simulink model "anti_interference"  (Simulink 7.2)
settings: Solver=ode45  StartTime=0.0  StopTime=0.02  RelTol=1e-3
undefined symbols (not defined in the file): get
libraries: dspbuff3 x24, dspxfrm3 x8, simulink x6, dspsigops x4, dspobslib x4, dspsnks4 x1
settings Model: Creator=Administrator  LastModifiedBy=Administrator

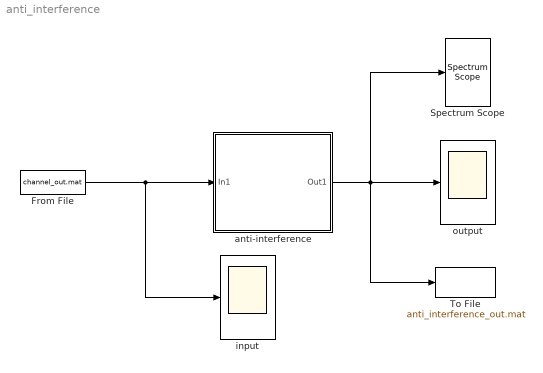
== system anti_interference ==
  From File : FromFile  FileName=channel_out.mat  SampleTime=1/5.1e6
  Spectrum Scope : dspsnks4/Spectrum Scope  DialogController=dspdialog.SpectrumScope  DialogControllerArgs=DataTag0  SystemSampleTime=-1  ScopeProperties=on  Domain=Frequency  HorizSpan=1  UseBuffer=on  BufferSize=2048  Overlap=64  inpFftLenInherit=off  FFTlength=128  numAvg=2  DisplayProperties=off  AxisGrid=on  Memory=off  FrameNumber=on  AxisLegend=off  AxisZoom=off  OpenScopeAtSimStart=on  OpenScopeImmediately=off  FigPos=get(0,'defaultfigureposition')  AxisProperties=off  XUnits=Hertz  XRange=[0...Fs/2]  XDisplay=0  InheritXIncr=on  XIncr=1.0  XLabel=Samples  XLimit=Auto  YUnits=dB  XMax=1  XMin=0  YLabel=Magnitude-squared, dB  LineProperties=off  wintypeSpecScope=Hann  RsSpecScope=50  betaSpecScope=5  winsampSpecScope=Periodic
      settings: YMin=-21.2867739282485  YMax=15.4884772920994
  To File : ToFile  Filename=anti_interference_out.mat
  anti-interference : Subsystem
  input : Scope
  output : Scope
  wires:
  From File/1 -> anti-interference/1(In1), input/1
  anti-interference/1(Out1) -> output/1, Spectrum Scope/1, To File/1

== system anti_interference/anti-interference ==
  In1 : Inport  OutDataType=sfix(16)  OutScaling=2^0
  Add1 : Sum  Inputs=++++  OutDataType=sfix(16)  OutScaling=2^-10
  Scope : Scope  NumInputPorts=5
      settings: YMin=-5~-5~-5~-5~-5  YMax=5~5~5~5~5  SaveName=ScopeData2
  firstroad : Subsystem
  fourthroad : Subsystem
  secondroad : Subsystem
  thirdroad : Subsystem
  Out1 : Outport  OutDataType=sfix(16)  OutScaling=2^0
  wires:
  firstroad/1(Out1) -> Add1/1, Scope/1
  secondroad/1(Out1) -> Add1/2, Scope/2
  thirdroad/1(Out1) -> Add1/3, Scope/3
  fourthroad/1(Out1) -> Add1/4, Scope/4
  In1/1 -> firstroad/1(In1), secondroad/1(In1), thirdroad/1(In1), fourthroad/1(In1)
  Add1/1 -> Out1/1, Scope/5

== system anti_interference/anti-interference/firstroad ==
  In1 : Inport  OutDataType=sfix(16)  OutScaling=2^0
  Complex to Magnitude-Angle : ComplexToMagnitudeAngle
  fft trans : Subsystem
  inteference_delieve : Subsystem
  inverse_convertion : Subsystem  Orientation=left
  threshold : Subsystem
  Out1 : Outport  Orientation=left  OutDataType=sfix(16)  OutScaling=2^0
  wires:
  fft trans/1(Out1) -> Complex to Magnitude-Angle/1
  Complex to Magnitude-Angle/1 -> threshold/1(In1), inteference_delieve/1(In1)
  Complex to Magnitude-Angle/2 -> inverse_convertion/1(In1)
  inteference_delieve/1(Out1) -> inverse_convertion/2(In2)
  threshold/1(Out1) -> inteference_delieve/2(In2)
  In1/1 -> fft trans/1(In1)
  inverse_convertion/1(Out1) -> Out1/1

== system anti_interference/anti-interference/fourthroad ==
  In1 : Inport  OutDataType=sfix(16)  OutScaling=2^0
  Complex to Magnitude-Angle : ComplexToMagnitudeAngle
  all : Subsystem
  inteference_delieve : Subsystem
  inverse_convertion : Subsystem  Orientation=left
  threshold : Subsystem
  Out1 : Outport  Orientation=left  OutDataType=sfix(16)  OutScaling=2^0
  wires:
  inverse_convertion/1(Out1) -> Out1/1
  In1/1 -> all/1(In1)
  threshold/1(Out1) -> inteference_delieve/2(In2)
  inteference_delieve/1(Out1) -> inverse_convertion/2(In2)
  Complex to Magnitude-Angle/2 -> inverse_convertion/1(In1)
  Complex to Magnitude-Angle/1 -> inteference_delieve/1(In1), threshold/1(In1)
  all/1(Out1) -> Complex to Magnitude-Angle/1

== system anti_interference/anti-interference/secondroad ==
  In1 : Inport  OutDataType=sfix(16)  OutScaling=2^0
  Complex to Magnitude-Angle : ComplexToMagnitudeAngle
  all : Subsystem
  inteference_delieve : Subsystem
  inverse_convertion : Subsystem  Orientation=left
  threshold : Subsystem
  Out1 : Outport  Orientation=left  OutDataType=sfix(16)  OutScaling=2^0
  wires:
  inverse_convertion/1(Out1) -> Out1/1
  In1/1 -> all/1(In1)
  threshold/1(Out1) -> inteference_delieve/2(In2)
  inteference_delieve/1(Out1) -> inverse_convertion/2(In2)
  Complex to Magnitude-Angle/2 -> inverse_convertion/1(In1)
  Complex to Magnitude-Angle/1 -> inteference_delieve/1(In1), threshold/1(In1)
  all/1(Out1) -> Complex to Magnitude-Angle/1

== system anti_interference/anti-interference/thirdroad ==
  In1 : Inport  OutDataType=sfix(16)  OutScaling=2^0
  Complex to Magnitude-Angle : ComplexToMagnitudeAngle
  all : Subsystem
  inteference_delieve : Subsystem
  inverse_convertion : Subsystem  Orientation=left
  threshold : Subsystem
  Out1 : Outport  Orientation=left  OutDataType=sfix(16)  OutScaling=2^0
  wires:
  all/1(Out1) -> Complex to Magnitude-Angle/1
  Complex to Magnitude-Angle/1 -> threshold/1(In1), inteference_delieve/1(In1)
  Complex to Magnitude-Angle/2 -> inverse_convertion/1(In1)
  inteference_delieve/1(Out1) -> inverse_convertion/2(In2)
  threshold/1(Out1) -> inteference_delieve/2(In2)
  In1/1 -> all/1(In1)
  inverse_convertion/1(Out1) -> Out1/1

== system anti_interference/anti-interference/firstroad/fft trans ==
  In1 : Inport  OutDataType=sfix(16)  OutScaling=2^0
  Buffer : dspbuff3/Buffer  N=8192  V=0  ic=0
  FFT1 : dspxfrm3/FFT  DialogController=dspDDGCreate  DialogControllerArgs=DataTag1  CompMethod=Table lookup  TableOpt=NEW  TableOptActive=Speed  BitRevOrder=off  InheritFFTLength=on  FFTLength=64  SkipNorm=off  roundingMode=Floor  overflowMode=off
  Window Function : dspsigops/Window Function  DialogController=dspDDGCreate  DialogControllerArgs=DataTag2  winmode=Apply window to input  wintype=Chebyshev  sampmode=Continuous  samptime=1  N=64  Rs=80  beta=10  winsamp=Symmetric  UserWindow=hamming  OptParams=off  UserParams={'symmetric'}  dataType=double  isSigned=on  wordLen=16  udDataType=sfix(16)  fracBitsMode=Best precision  numFracBits=15  roundingMode=Floor  overflowMode=off  numSidelobes=4  sidelobeLevel=-30
  Out1 : Outport  OutDataType=sfix(16)  OutScaling=2^0
  wires:
  Buffer/1 -> Window Function/1
  FFT1/1 -> Out1/1
  In1/1 -> Buffer/1
  Window Function/1 -> FFT1/1

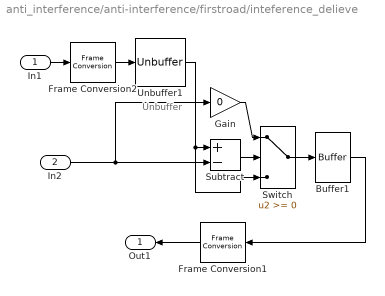
== system anti_interference/anti-interference/firstroad/inteference_delieve ==
  note: Unbuffer
  In1 : Inport  OutDataType=sfix(16)  OutScaling=2^0
  In2 : Inport  Port=2  OutDataType=sfix(16)  OutScaling=2^0
  Buffer1 : dspbuff3/Buffer  N=8192  V=0  ic=0
  Frame Conversion1 : FrameConversion  Orientation=left  OutFrame=Sample-based
  Frame Conversion2 : FrameConversion
  Gain : Gain  Gain=0  ParameterDataType=sfix(16)  ParameterScaling=2^0  OutDataType=sfix(16)  OutScaling=2^0
  Subtract : Sum  Inputs=+-  OutDataType=sfix(16)  OutScaling=2^-10
  Switch : Switch
  Unbuffer1 : dspbuff3/Unbuffer  ic=0
  Out1 : Outport  Orientation=left  OutDataType=sfix(16)  OutScaling=2^0
  wires:
  Unbuffer1/1 -> Subtract/1, Switch/3
  In2/1 -> Subtract/2, Gain/1
  Subtract/1 -> Switch/2
  Gain/1 -> Switch/1
  Switch/1 -> Buffer1/1
  In1/1 -> Frame Conversion2/1
  Frame Conversion2/1 -> Unbuffer1/1
  Frame Conversion1/1 -> Out1/1
  Buffer1/1 -> Frame Conversion1/1

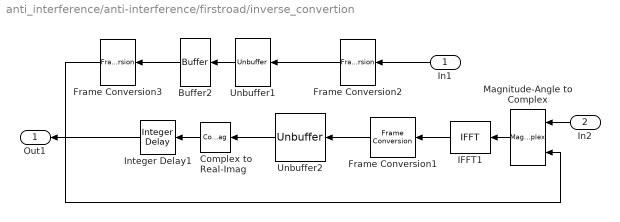
== system anti_interference/anti-interference/firstroad/inverse_convertion ==
  In1 : Inport  Orientation=left  OutDataType=sfix(16)  OutScaling=2^0
  In2 : Inport  Orientation=left  Port=2  OutDataType=sfix(16)  OutScaling=2^0
  Buffer2 : dspbuff3/Buffer  Orientation=left  N=8192  V=0  ic=0
  Complex to Real-Imag : ComplexToRealImag  Orientation=left  Output=Real
  Frame Conversion1 : FrameConversion  Orientation=left
  Frame Conversion2 : FrameConversion  Orientation=left
  Frame Conversion3 : FrameConversion  Orientation=left  OutFrame=Sample-based
  IFFT1 : dspxfrm3/IFFT  Orientation=left  DialogController=dspDDGCreate  DialogControllerArgs=DataTag3  CompMethod=Table lookup  TableOpt=NEW  TableOptActive=Speed  BitRevOrder=off  cs_in=off  SkipNorm=on  InheritFFTLength=on  FFTLength=64  mode=Complex  outSamplingMode=Sample based  roundingMode=Floor  overflowMode=off
  Integer Delay1 : simulink/Discrete/Integer Delay  Orientation=left  vinit=0.0  samptime=-1  NumDelays=6144
  Magnitude-Angle to Complex : MagnitudeAngleToComplex  Orientation=left
  Unbuffer1 : dspbuff3/Unbuffer  Orientation=left  ic=0
  Unbuffer2 : dspbuff3/Unbuffer  Orientation=left  ic=0
  Out1 : Outport  Orientation=left  OutDataType=sfix(16)  OutScaling=2^0
  wires:
  Frame Conversion2/1 -> Unbuffer1/1
  Unbuffer1/1 -> Buffer2/1
  Buffer2/1 -> Frame Conversion3/1
  Magnitude-Angle to Complex/1 -> IFFT1/1
  Unbuffer2/1 -> Complex to Real-Imag/1
  Frame Conversion3/1 -> Magnitude-Angle to Complex/2
  Complex to Real-Imag/1 -> Integer Delay1/1
  In1/1 -> Frame Conversion2/1
  In2/1 -> Magnitude-Angle to Complex/1
  IFFT1/1 -> Frame Conversion1/1
  Frame Conversion1/1 -> Unbuffer2/1
  Integer Delay1/1 -> Out1/1

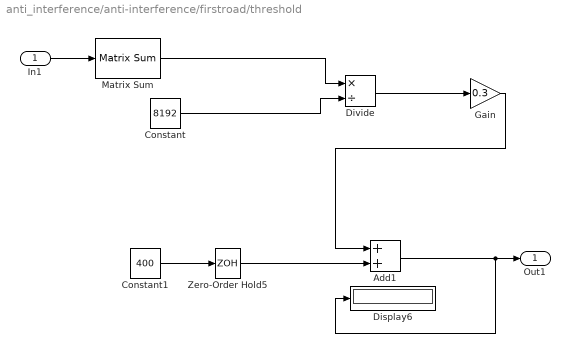
== system anti_interference/anti-interference/firstroad/threshold ==
  In1 : Inport  OutDataType=sfix(16)  OutScaling=2^0
  Add1 : Sum  OutDataType=sfix(16)  OutScaling=2^-10
  Constant : Constant  Value=8192  OutDataType=sfix(16)  OutScaling=2^0
  Constant1 : Constant  Value=400  OutDataType=sfix(16)  OutScaling=2^0
  Display6 : Display
  Divide : Product  Inputs=*/  OutDataType=sfix(16)  OutScaling=2^-10
  Gain : Gain  Gain=0.3  ParameterDataType=sfix(16)  ParameterScaling=2^0  OutDataType=sfix(16)  OutScaling=2^0
  Matrix Sum : dspobslib/Matrix Sum  DialogController=dspDDGCreate  DialogControllerArgs=DataTag4  Dim=Columns  roundingMode=Floor  overflowMode=off
  Zero-Order Hold5 : ZeroOrderHold  SampleTime=1/5.1e6
  Out1 : Outport  OutDataType=sfix(16)  OutScaling=2^0
  wires:
  Matrix Sum/1 -> Divide/1
  Divide/1 -> Gain/1
  Gain/1 -> Add1/1
  Add1/1 -> Display6/1, Out1/1
  In1/1 -> Matrix Sum/1
  Constant1/1 -> Zero-Order Hold5/1
  Constant/1 -> Divide/2
  Zero-Order Hold5/1 -> Add1/2

== system anti_interference/anti-interference/fourthroad/all ==
  In1 : Inport  OutDataType=sfix(16)  OutScaling=2^0
  Buffer1 : dspbuff3/Buffer  N=8192  V=0  ic=0
  FFT : dspxfrm3/FFT  DialogController=dspDDGCreate  DialogControllerArgs=DataTag5  CompMethod=Table lookup  TableOpt=NEW  TableOptActive=Speed  BitRevOrder=off  InheritFFTLength=on  FFTLength=64  SkipNorm=off  roundingMode=Floor  overflowMode=off
  Integer Delay : simulink/Discrete/Integer Delay  vinit=0.0  samptime=-1  NumDelays=6144
  Window Function1 : dspsigops/Window Function  DialogController=dspDDGCreate  DialogControllerArgs=DataTag6  winmode=Apply window to input  wintype=Chebyshev  sampmode=Continuous  samptime=1  N=64  Rs=80  beta=10  winsamp=Symmetric  UserWindow=hamming  OptParams=off  UserParams={'symmetric'}  dataType=double  isSigned=on  wordLen=16  udDataType=sfix(16)  fracBitsMode=Best precision  numFracBits=15  roundingMode=Floor  overflowMode=off  numSidelobes=4  sidelobeLevel=-30
  Out1 : Outport  OutDataType=sfix(16)  OutScaling=2^0
  wires:
  In1/1 -> Buffer1/1
  Buffer1/1 -> Integer Delay/1
  Integer Delay/1 -> Window Function1/1
  Window Function1/1 -> FFT/1
  FFT/1 -> Out1/1

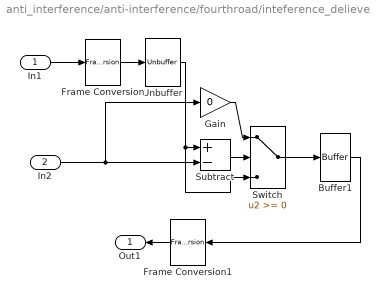
== system anti_interference/anti-interference/fourthroad/inteference_delieve ==
  In1 : Inport  OutDataType=sfix(16)  OutScaling=2^0
  In2 : Inport  Port=2  OutDataType=sfix(16)  OutScaling=2^0
  Buffer1 : dspbuff3/Buffer  N=8192  V=0  ic=0
  Frame Conversion : FrameConversion
  Frame Conversion1 : FrameConversion  Orientation=left  OutFrame=Sample-based
  Gain : Gain  Gain=0  ParameterDataType=sfix(16)  ParameterScaling=2^0  OutDataType=sfix(16)  OutScaling=2^0
  Subtract : Sum  Inputs=+-  OutDataType=sfix(16)  OutScaling=2^-10
  Switch : Switch
  Unbuffer : dspbuff3/Unbuffer  ic=0
  Out1 : Outport  Orientation=left  OutDataType=sfix(16)  OutScaling=2^0
  wires:
  Frame Conversion1/1 -> Out1/1
  In1/1 -> Frame Conversion/1
  Buffer1/1 -> Frame Conversion1/1
  Switch/1 -> Buffer1/1
  Gain/1 -> Switch/1
  Subtract/1 -> Switch/2
  In2/1 -> Gain/1, Subtract/2
  Frame Conversion/1 -> Unbuffer/1
  Unbuffer/1 -> Switch/3, Subtract/1

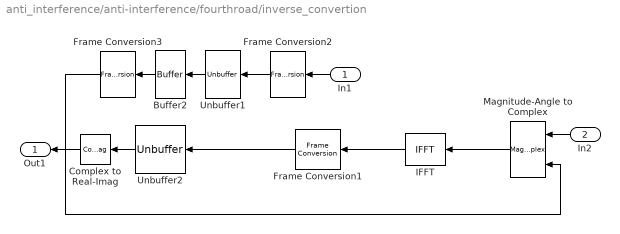
== system anti_interference/anti-interference/fourthroad/inverse_convertion ==
  In1 : Inport  Orientation=left  OutDataType=sfix(16)  OutScaling=2^0
  In2 : Inport  Orientation=left  Port=2  OutDataType=sfix(16)  OutScaling=2^0
  Buffer2 : dspbuff3/Buffer  Orientation=left  N=8192  V=0  ic=0
  Complex to Real-Imag : ComplexToRealImag  Orientation=left  Output=Real
  Frame Conversion1 : FrameConversion  Orientation=left
  Frame Conversion2 : FrameConversion  Orientation=left
  Frame Conversion3 : FrameConversion  Orientation=left  OutFrame=Sample-based
  IFFT : dspxfrm3/IFFT  Orientation=left  DialogController=dspDDGCreate  DialogControllerArgs=DataTag7  CompMethod=Table lookup  TableOpt=NEW  TableOptActive=Speed  BitRevOrder=off  cs_in=off  SkipNorm=on  InheritFFTLength=on  FFTLength=64  mode=Complex  outSamplingMode=Sample based  roundingMode=Floor  overflowMode=off
  Magnitude-Angle to Complex : MagnitudeAngleToComplex  Orientation=left
  Unbuffer1 : dspbuff3/Unbuffer  Orientation=left  ic=0
  Unbuffer2 : dspbuff3/Unbuffer  Orientation=left  ic=0
  Out1 : Outport  Orientation=left  OutDataType=sfix(16)  OutScaling=2^0
  wires:
  In2/1 -> Magnitude-Angle to Complex/1
  In1/1 -> Frame Conversion2/1
  Complex to Real-Imag/1 -> Out1/1
  Frame Conversion3/1 -> Magnitude-Angle to Complex/2
  Unbuffer2/1 -> Complex to Real-Imag/1
  Magnitude-Angle to Complex/1 -> IFFT/1
  Buffer2/1 -> Frame Conversion3/1
  Unbuffer1/1 -> Buffer2/1
  Frame Conversion2/1 -> Unbuffer1/1
  IFFT/1 -> Frame Conversion1/1
  Frame Conversion1/1 -> Unbuffer2/1

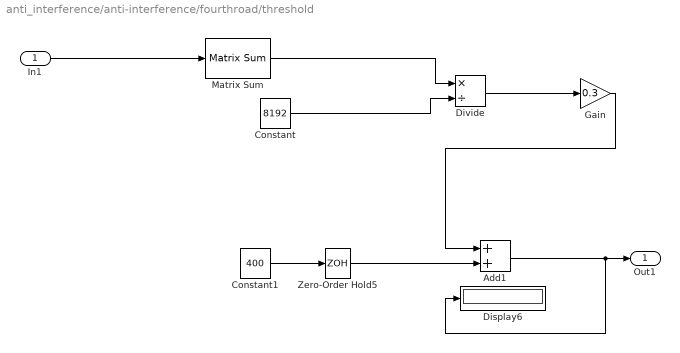
== system anti_interference/anti-interference/fourthroad/threshold ==
  In1 : Inport  OutDataType=sfix(16)  OutScaling=2^0
  Add1 : Sum  OutDataType=sfix(16)  OutScaling=2^-10
  Constant : Constant  Value=8192  OutDataType=sfix(16)  OutScaling=2^0
  Constant1 : Constant  Value=400  OutDataType=sfix(16)  OutScaling=2^0
  Display6 : Display
  Divide : Product  Inputs=*/  OutDataType=sfix(16)  OutScaling=2^-10
  Gain : Gain  Gain=0.3  ParameterDataType=sfix(16)  ParameterScaling=2^0  OutDataType=sfix(16)  OutScaling=2^0
  Matrix Sum : dspobslib/Matrix Sum  DialogController=dspDDGCreate  DialogControllerArgs=DataTag8  Dim=Columns  roundingMode=Floor  overflowMode=off
  Zero-Order Hold5 : ZeroOrderHold  SampleTime=1/5.1e6
  Out1 : Outport  OutDataType=sfix(16)  OutScaling=2^0
  wires:
  Zero-Order Hold5/1 -> Add1/2
  Constant/1 -> Divide/2
  Constant1/1 -> Zero-Order Hold5/1
  In1/1 -> Matrix Sum/1
  Add1/1 -> Out1/1, Display6/1
  Gain/1 -> Add1/1
  Divide/1 -> Gain/1
  Matrix Sum/1 -> Divide/1

== system anti_interference/anti-interference/secondroad/all ==
  In1 : Inport  OutDataType=sfix(16)  OutScaling=2^0
  Buffer1 : dspbuff3/Buffer  N=8192  V=0  ic=0
  FFT : dspxfrm3/FFT  DialogController=dspDDGCreate  DialogControllerArgs=DataTag9  CompMethod=Table lookup  TableOpt=NEW  TableOptActive=Speed  BitRevOrder=off  InheritFFTLength=on  FFTLength=64  SkipNorm=off  roundingMode=Floor  overflowMode=off
  Integer Delay : simulink/Discrete/Integer Delay  vinit=0.0  samptime=-1  NumDelays=2048
  Window Function1 : dspsigops/Window Function  DialogController=dspDDGCreate  DialogControllerArgs=DataTag10  winmode=Apply window to input  wintype=Chebyshev  sampmode=Continuous  samptime=1  N=64  Rs=80  beta=10  winsamp=Symmetric  UserWindow=hamming  OptParams=off  UserParams={'symmetric'}  dataType=double  isSigned=on  wordLen=16  udDataType=sfix(16)  fracBitsMode=Best precision  numFracBits=15  roundingMode=Floor  overflowMode=off  numSidelobes=4  sidelobeLevel=-30
  Out1 : Outport  OutDataType=sfix(16)  OutScaling=2^0
  wires:
  In1/1 -> Buffer1/1
  Buffer1/1 -> Integer Delay/1
  Integer Delay/1 -> Window Function1/1
  Window Function1/1 -> FFT/1
  FFT/1 -> Out1/1

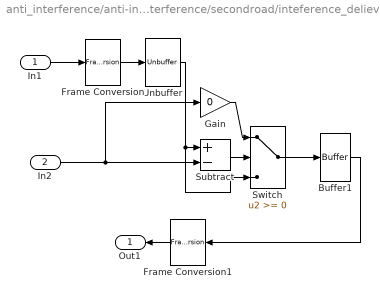
== system anti_interference/anti-interference/secondroad/inteference_delieve ==
  In1 : Inport  OutDataType=sfix(16)  OutScaling=2^0
  In2 : Inport  Port=2  OutDataType=sfix(16)  OutScaling=2^0
  Buffer1 : dspbuff3/Buffer  N=8192  V=0  ic=0
  Frame Conversion : FrameConversion
  Frame Conversion1 : FrameConversion  Orientation=left  OutFrame=Sample-based
  Gain : Gain  Gain=0  ParameterDataType=sfix(16)  ParameterScaling=2^0  OutDataType=sfix(16)  OutScaling=2^0
  Subtract : Sum  Inputs=+-  OutDataType=sfix(16)  OutScaling=2^-10
  Switch : Switch
  Unbuffer : dspbuff3/Unbuffer  ic=0
  Out1 : Outport  Orientation=left  OutDataType=sfix(16)  OutScaling=2^0
  wires:
  Frame Conversion1/1 -> Out1/1
  In1/1 -> Frame Conversion/1
  Buffer1/1 -> Frame Conversion1/1
  Switch/1 -> Buffer1/1
  Gain/1 -> Switch/1
  Subtract/1 -> Switch/2
  In2/1 -> Gain/1, Subtract/2
  Frame Conversion/1 -> Unbuffer/1
  Unbuffer/1 -> Switch/3, Subtract/1

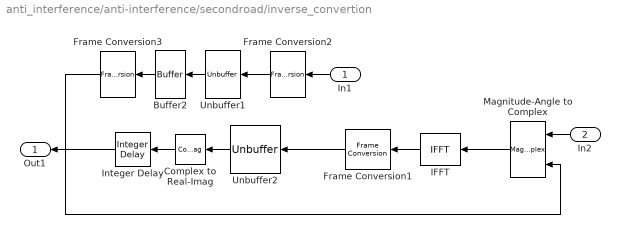
== system anti_interference/anti-interference/secondroad/inverse_convertion ==
  In1 : Inport  Orientation=left  OutDataType=sfix(16)  OutScaling=2^0
  In2 : Inport  Orientation=left  Port=2  OutDataType=sfix(16)  OutScaling=2^0
  Buffer2 : dspbuff3/Buffer  Orientation=left  N=8192  V=0  ic=0
  Complex to Real-Imag : ComplexToRealImag  Orientation=left  Output=Real
  Frame Conversion1 : FrameConversion  Orientation=left
  Frame Conversion2 : FrameConversion  Orientation=left
  Frame Conversion3 : FrameConversion  Orientation=left  OutFrame=Sample-based
  IFFT : dspxfrm3/IFFT  Orientation=left  DialogController=dspDDGCreate  DialogControllerArgs=DataTag11  CompMethod=Table lookup  TableOpt=NEW  TableOptActive=Speed  BitRevOrder=off  cs_in=off  SkipNorm=on  InheritFFTLength=on  FFTLength=64  mode=Complex  outSamplingMode=Sample based  roundingMode=Floor  overflowMode=off
  Integer Delay : simulink/Discrete/Integer Delay  Orientation=left  vinit=0.0  samptime=-1  NumDelays=4096
  Magnitude-Angle to Complex : MagnitudeAngleToComplex  Orientation=left
  Unbuffer1 : dspbuff3/Unbuffer  Orientation=left  ic=0
  Unbuffer2 : dspbuff3/Unbuffer  Orientation=left  ic=0
  Out1 : Outport  Orientation=left  OutDataType=sfix(16)  OutScaling=2^0
  wires:
  In2/1 -> Magnitude-Angle to Complex/1
  In1/1 -> Frame Conversion2/1
  Complex to Real-Imag/1 -> Integer Delay/1
  Frame Conversion3/1 -> Magnitude-Angle to Complex/2
  Unbuffer2/1 -> Complex to Real-Imag/1
  Magnitude-Angle to Complex/1 -> IFFT/1
  Buffer2/1 -> Frame Conversion3/1
  Unbuffer1/1 -> Buffer2/1
  Frame Conversion2/1 -> Unbuffer1/1
  IFFT/1 -> Frame Conversion1/1
  Frame Conversion1/1 -> Unbuffer2/1
  Integer Delay/1 -> Out1/1

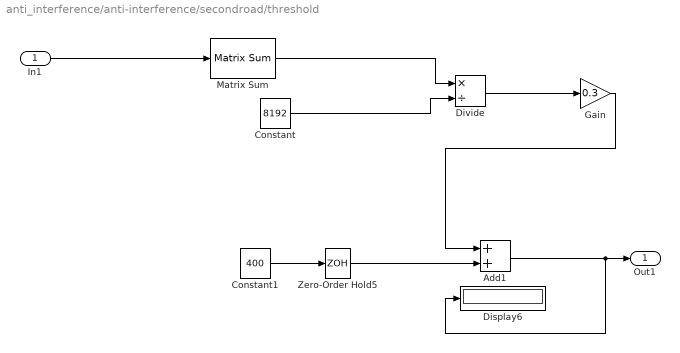
== system anti_interference/anti-interference/secondroad/threshold ==
  In1 : Inport  OutDataType=sfix(16)  OutScaling=2^0
  Add1 : Sum  OutDataType=sfix(16)  OutScaling=2^-10
  Constant : Constant  Value=8192  OutDataType=sfix(16)  OutScaling=2^0
  Constant1 : Constant  Value=400  OutDataType=sfix(16)  OutScaling=2^0
  Display6 : Display
  Divide : Product  Inputs=*/  OutDataType=sfix(16)  OutScaling=2^-10
  Gain : Gain  Gain=0.3  ParameterDataType=sfix(16)  ParameterScaling=2^0  OutDataType=sfix(16)  OutScaling=2^0
  Matrix Sum : dspobslib/Matrix Sum  DialogController=dspDDGCreate  DialogControllerArgs=DataTag12  Dim=Columns  roundingMode=Floor  overflowMode=off
  Zero-Order Hold5 : ZeroOrderHold  SampleTime=1/5.1e6
  Out1 : Outport  OutDataType=sfix(16)  OutScaling=2^0
  wires:
  Zero-Order Hold5/1 -> Add1/2
  Constant/1 -> Divide/2
  Constant1/1 -> Zero-Order Hold5/1
  In1/1 -> Matrix Sum/1
  Add1/1 -> Out1/1, Display6/1
  Gain/1 -> Add1/1
  Divide/1 -> Gain/1
  Matrix Sum/1 -> Divide/1

== system anti_interference/anti-interference/thirdroad/all ==
  In1 : Inport  OutDataType=sfix(16)  OutScaling=2^0
  Buffer1 : dspbuff3/Buffer  N=8192  V=0  ic=0
  FFT : dspxfrm3/FFT  DialogController=dspDDGCreate  DialogControllerArgs=DataTag13  CompMethod=Table lookup  TableOpt=NEW  TableOptActive=Speed  BitRevOrder=off  InheritFFTLength=on  FFTLength=64  SkipNorm=off  roundingMode=Floor  overflowMode=off
  Integer Delay : simulink/Discrete/Integer Delay  vinit=0.0  samptime=-1  NumDelays=4096
  Window Function1 : dspsigops/Window Function  DialogController=dspDDGCreate  DialogControllerArgs=DataTag14  winmode=Apply window to input  wintype=Chebyshev  sampmode=Continuous  samptime=1  N=64  Rs=80  beta=10  winsamp=Symmetric  UserWindow=hamming  OptParams=off  UserParams={'symmetric'}  dataType=double  isSigned=on  wordLen=16  udDataType=sfix(16)  fracBitsMode=Best precision  numFracBits=15  roundingMode=Floor  overflowMode=off  numSidelobes=4  sidelobeLevel=-30
  Out1 : Outport  OutDataType=sfix(16)  OutScaling=2^0
  wires:
  In1/1 -> Buffer1/1
  Buffer1/1 -> Integer Delay/1
  Integer Delay/1 -> Window Function1/1
  Window Function1/1 -> FFT/1
  FFT/1 -> Out1/1

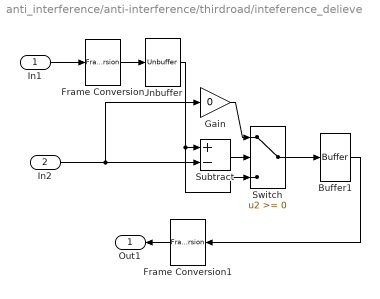
== system anti_interference/anti-interference/thirdroad/inteference_delieve ==
  In1 : Inport  OutDataType=sfix(16)  OutScaling=2^0
  In2 : Inport  Port=2  OutDataType=sfix(16)  OutScaling=2^0
  Buffer1 : dspbuff3/Buffer  N=8192  V=0  ic=0
  Frame Conversion : FrameConversion
  Frame Conversion1 : FrameConversion  Orientation=left  OutFrame=Sample-based
  Gain : Gain  Gain=0  ParameterDataType=sfix(16)  ParameterScaling=2^0  OutDataType=sfix(16)  OutScaling=2^0
  Subtract : Sum  Inputs=+-  OutDataType=sfix(16)  OutScaling=2^-10
  Switch : Switch
  Unbuffer : dspbuff3/Unbuffer  ic=0
  Out1 : Outport  Orientation=left  OutDataType=sfix(16)  OutScaling=2^0
  wires:
  Unbuffer/1 -> Subtract/1, Switch/3
  Frame Conversion/1 -> Unbuffer/1
  In2/1 -> Subtract/2, Gain/1
  Subtract/1 -> Switch/2
  Gain/1 -> Switch/1
  Switch/1 -> Buffer1/1
  Buffer1/1 -> Frame Conversion1/1
  In1/1 -> Frame Conversion/1
  Frame Conversion1/1 -> Out1/1

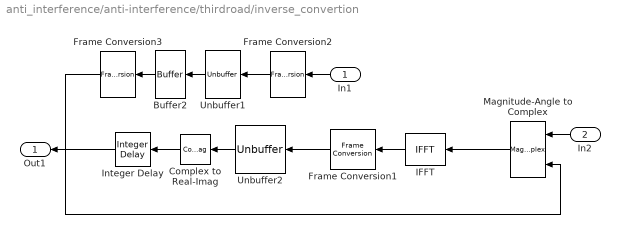
== system anti_interference/anti-interference/thirdroad/inverse_convertion ==
  In1 : Inport  Orientation=left  OutDataType=sfix(16)  OutScaling=2^0
  In2 : Inport  Orientation=left  Port=2  OutDataType=sfix(16)  OutScaling=2^0
  Buffer2 : dspbuff3/Buffer  Orientation=left  N=8192  V=0  ic=0
  Complex to Real-Imag : ComplexToRealImag  Orientation=left  Output=Real
  Frame Conversion1 : FrameConversion  Orientation=left
  Frame Conversion2 : FrameConversion  Orientation=left
  Frame Conversion3 : FrameConversion  Orientation=left  OutFrame=Sample-based
  IFFT : dspxfrm3/IFFT  Orientation=left  DialogController=dspDDGCreate  DialogControllerArgs=DataTag15  CompMethod=Table lookup  TableOpt=NEW  TableOptActive=Speed  BitRevOrder=off  cs_in=off  SkipNorm=on  InheritFFTLength=on  FFTLength=64  mode=Complex  outSamplingMode=Sample based  roundingMode=Floor  overflowMode=off
  Integer Delay : simulink/Discrete/Integer Delay  Orientation=left  vinit=0.0  samptime=-1  NumDelays=2048
  Magnitude-Angle to Complex : MagnitudeAngleToComplex  Orientation=left
  Unbuffer1 : dspbuff3/Unbuffer  Orientation=left  ic=0
  Unbuffer2 : dspbuff3/Unbuffer  Orientation=left  ic=0
  Out1 : Outport  Orientation=left  OutDataType=sfix(16)  OutScaling=2^0
  wires:
  Frame Conversion2/1 -> Unbuffer1/1
  Unbuffer1/1 -> Buffer2/1
  Buffer2/1 -> Frame Conversion3/1
  Magnitude-Angle to Complex/1 -> IFFT/1
  Unbuffer2/1 -> Complex to Real-Imag/1
  Frame Conversion3/1 -> Magnitude-Angle to Complex/2
  Complex to Real-Imag/1 -> Integer Delay/1
  In1/1 -> Frame Conversion2/1
  In2/1 -> Magnitude-Angle to Complex/1
  IFFT/1 -> Frame Conversion1/1
  Frame Conversion1/1 -> Unbuffer2/1
  Integer Delay/1 -> Out1/1

== system anti_interference/anti-interference/thirdroad/threshold ==
  In1 : Inport  OutDataType=sfix(16)  OutScaling=2^0
  Add1 : Sum  OutDataType=sfix(16)  OutScaling=2^-10
  Constant : Constant  Value=8192  OutDataType=sfix(16)  OutScaling=2^0
  Constant1 : Constant  Value=400  OutDataType=sfix(16)  OutScaling=2^0
  Display6 : Display
  Divide : Product  Inputs=*/  OutDataType=sfix(16)  OutScaling=2^-10
  Gain : Gain  Gain=0.3  ParameterDataType=sfix(16)  ParameterScaling=2^0  OutDataType=sfix(16)  OutScaling=2^0
  Matrix Sum : dspobslib/Matrix Sum  DialogController=dspDDGCreate  DialogControllerArgs=DataTag16  Dim=Columns  roundingMode=Floor  overflowMode=off
  Zero-Order Hold5 : ZeroOrderHold  SampleTime=1/5.1e6
  Out1 : Outport  OutDataType=sfix(16)  OutScaling=2^0
  wires:
  Matrix Sum/1 -> Divide/1
  Divide/1 -> Gain/1
  Gain/1 -> Add1/1
  Add1/1 -> Display6/1, Out1/1
  In1/1 -> Matrix Sum/1
  Constant1/1 -> Zero-Order Hold5/1
  Constant/1 -> Divide/2
  Zero-Order Hold5/1 -> Add1/2
